simulink model "full_model_feedbackLinearization"  (R2022a)
settings: Solver=VariableStepAuto  StartTime=0.0  StopTime=t_end  FixedStep=1e-4  RelTol=1e-9  AbsTol=1e-9
undefined symbols (not defined in the file): hControl, omega_0, paramStruct, theta_0
settings Model: PauseTimes=0  Creator=Philipp  LastModifiedBy=Philipp
settings DebuggingCC: UnconnectedInputMsg=warning  UnconnectedOutputMsg=warning  UnconnectedLineMsg=warning  UnderSpecifiedDimensionMsg=warning
settings ModelReferenceCC: ModelReferenceMinAlgLoopOccurrences=on
settings RTWCC: DLArmComputeVersion=19.05

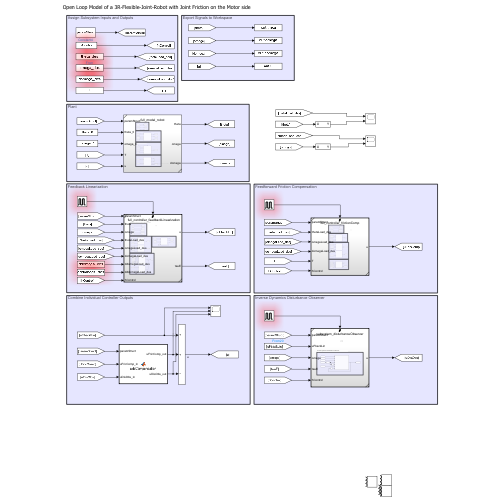
[thumbnail: Simulink's stored preview of the top-level diagram]
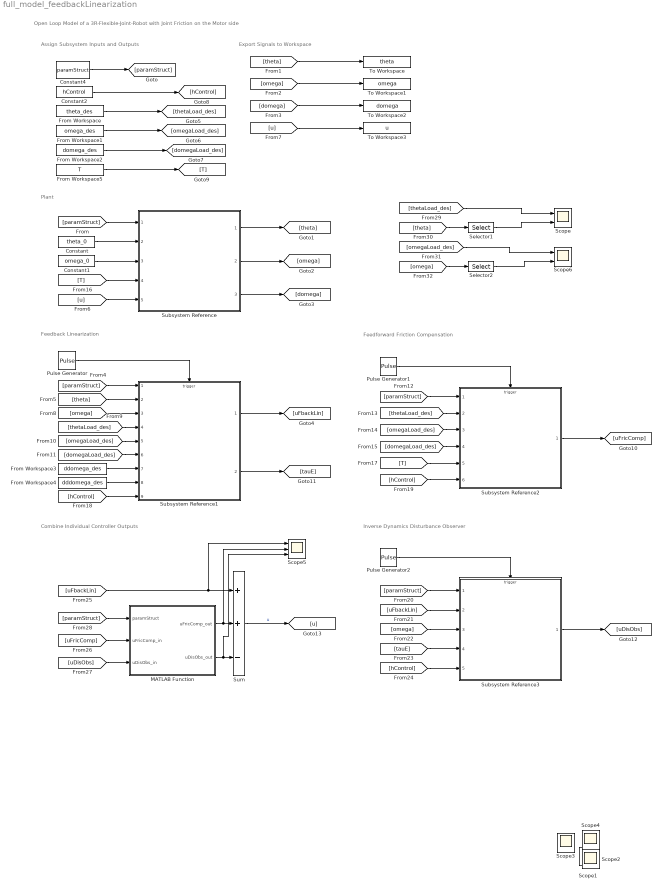
== system full_model_feedbackLinearization ==
  note: Feedback Linearization
  note: Export Signals to Workspace
  note: Plant
  note: Open Loop Model of a 3R-Flexible-Joint-Robot with Joint Friction on the Motor side
  note: Feedforward Friction Compensation
  note: Inverse Dynamics Disturbance Observer
  note: Combine Individual Controller Outputs
  note: Assign Subsystem Inputs and Outputs
  Constant : Constant  Value=theta_0
  Constant1 : Constant  Value=omega_0
  Constant2 : Constant  Value=hControl
  Constant4 : Constant  InitFcn=|  Value=paramStruct  OutDataTypeStr=Bus: main_bus
      | % Import MATLAB evalin command
      | eml.extrinsic('evalin');
      | 
      | 
      | % Get contents of the structure a and output it
      | y = evalin('base', 'paramStruct');
  From Workspace : FromWorkspace  VariableName=theta_des
  From Workspace1 : FromWorkspace  VariableName=omega_des
  From Workspace2 : FromWorkspace  VariableName=domega_des
  From Workspace3 : FromWorkspace  VariableName=ddomega_des
  From Workspace4 : FromWorkspace  VariableName=dddomega_des
  From Workspace5 : FromWorkspace  VariableName=T
  MATLAB Function : MATLAB Function  TreatAsAtomicUnit=on
  Pulse Generator : DiscretePulseGenerator  PulseType=Time based  Period=hControl  PulseWidth=5
  Pulse Generator1 : DiscretePulseGenerator  PulseType=Time based  Period=hControl  PulseWidth=5
  Pulse Generator2 : DiscretePulseGenerator  PulseType=Time based  Period=hControl  PulseWidth=5
  Scope : Scope  NumInputPorts=2
  Scope{1..5} (5 alike) : Scope  NumInputPorts=3
  Scope6 : Scope  NumInputPorts=2
  Selector1 : Selector  InputPortWidth=6  IndexOptions=Index vector (dialog)  Indices=1:3  OutputSizes=1
  Selector2 : Selector  InputPortWidth=6  IndexOptions=Index vector (dialog)  Indices=1:3  OutputSizes=1
  Subsystem Reference : Subsystem  ReferencedSubsystem=full_model_robot
  Subsystem Reference1 : Subsystem  ReferencedSubsystem=full_controller_feedbackLinearization
  Subsystem Reference2 : Subsystem  ReferencedSubsystem=full_controller_frictionComp
  Subsystem Reference3 : Subsystem  ReferencedSubsystem=subsystem_disturbanceObserver
  Sum : Sum  Inputs=++-
  To Workspace : ToWorkspace  VariableName=theta  SampleTime=-1
  To Workspace1 : ToWorkspace  VariableName=omega  SampleTime=-1
  To Workspace2 : ToWorkspace  VariableName=domega  SampleTime=-1
  To Workspace3 : ToWorkspace  VariableName=u  SampleTime=-1
  wires:
  Constant/1 -> Subsystem Reference/2
  Constant1/1 -> Subsystem Reference/3
  [paramStruct] -> Subsystem Reference/1
  Subsystem Reference/1 -> [theta]
  Subsystem Reference/2 -> [omega]
  Subsystem Reference/3 -> [domega]
  [theta] -> To Workspace/1
  [domega] -> To Workspace2/1
  [omega] -> To Workspace1/1
  Constant4/1 -> [paramStruct]
  [paramStruct] -> Subsystem Reference1/1
  [theta] -> Subsystem Reference1/2
  [u] -> To Workspace3/1
  [u] -> Subsystem Reference/5
  [omega] -> Subsystem Reference1/3
  From Workspace/1 -> [thetaLoad_des]
  From Workspace1/1 -> [omegaLoad_des]
  From Workspace2/1 -> [domegaLoad_des]
  From Workspace3/1 -> Subsystem Reference1/7
  From Workspace4/1 -> Subsystem Reference1/8
  Constant2/1 -> [hControl]
  [thetaLoad_des] -> Subsystem Reference1/4
  [omegaLoad_des] -> Subsystem Reference1/5
  [domegaLoad_des] -> Subsystem Reference1/6
  Pulse Generator/1 -> Subsystem Reference1/Trigger
  Pulse Generator1/1 -> Subsystem Reference2/Trigger
  [paramStruct] -> Subsystem Reference2/1
  [thetaLoad_des] -> Subsystem Reference2/2
  [omegaLoad_des] -> Subsystem Reference2/3
  [domegaLoad_des] -> Subsystem Reference2/4
  [T] -> Subsystem Reference/4
  [T] -> Subsystem Reference2/5
  [hControl] -> Subsystem Reference1/9
  [hControl] -> Subsystem Reference2/6
  Subsystem Reference2/1 -> [uFricComp]
  Pulse Generator2/1 -> Subsystem Reference3/Trigger
  [paramStruct] -> Subsystem Reference3/1
  [uFbackLin] -> Subsystem Reference3/2
  [omega] -> Subsystem Reference3/3
  [tauE] -> Subsystem Reference3/4
  Subsystem Reference1/2 -> [tauE]
  [hControl] -> Subsystem Reference3/5
  Subsystem Reference3/1 -> [uDisObs]
  MATLAB Function/2(uDisObs_out) -> Scope5/3, Sum/3
  MATLAB Function/1(uFricComp_out) -> Scope5/2, Sum/2
  [uDisObs] -> MATLAB Function/3(uDisObs_in)
  [uFricComp] -> MATLAB Function/2(uFricComp_in)
  [uFbackLin] -> Scope5/1, Sum/1
  [paramStruct] -> MATLAB Function/1(paramStruct)
  Sum/1 -> [u]  "u"
  Subsystem Reference1/1 -> [uFbackLin]
  From Workspace5/1 -> [T]
  [theta] -> Selector1/1
  [thetaLoad_des] -> Scope/1
  Selector1/1 -> Scope/2
  [omega] -> Selector2/1
  [omegaLoad_des] -> Scope6/1
  Selector2/1 -> Scope6/2

== matlab function full_model_feedbackLinearization/MATLAB Function ==
  data: paramStruct input; uFricComp_out output; uFricComp_in input; uDisObs_in input; uDisObs_out output
function [uFricComp_out, uDisObs_out] = addCompensation(paramStruct, uFricComp_in, uDisObs_in)

uFricComp_out = zeros(3,1);
uDisObs_out = zeros(3,1);

if paramStruct.feedbackLinearization.addFrictionComp
    uFricComp_out = uFricComp_in;
end
if paramStruct.feedbackLinearization.addDisturbanceObs
    uDisObs_out = uDisObs_in;
end
